simulink model "if_and_if_action_subsys"  (R2014a)
settings: Solver=FixedStepDiscrete  StartTime=0.0  StopTime=10.0  FixedStep=0.1  RelTol=1e-3
settings Model: BufferReuse=off  Creator=yoshi12  LastModifiedBy=ts1413
settings OptimizationCC: BlockReduction=off  OptimizeBlockIOStorage=off  BufferReuse=off  GlobalBufferReuse=off  ExpressionFolding=off  LocalBlockOutputs=off  OptimizeModelRefInitCode=on  LifeSpan=1
settings RTWCC: SystemTargetFile=ert.tlc  GenCodeOnly=on  TemplateMakefile=ert_default_tmf  Description=Embedded Coder  ProcessScript=ert_make_rtw_hook
settings CodeAppCC: IgnoreCustomStorageClasses=off
settings ERTTargetCC: ParMdlRefBuildCompliant=on  CompOptLevelCompliant=on  ConcurrentExecutionCompliant=on  ERTFirstTimeCompliant=on  ModelStepFunctionPrototypeControlCompliant=on  CPPClassGenCompliant=on  InlinedParameterPlacement=Hierarchical  ERTCustomFileTemplate=example_file_process.tlc

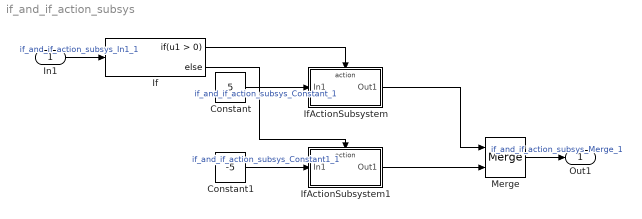
== system if_and_if_action_subsys ==
  In1 : Inport
  Constant : Constant  Value=5
  Constant1 : Constant  Value=-5
  If : If
  IfActionSubsystem : Subsystem  TreatAsAtomicUnit=on
  IfActionSubsystem1 : Subsystem  TreatAsAtomicUnit=on
  Merge : Merge  InitialOutput=0
  Out1 : Outport
  wires:
  In1/1 -> If/1  "if_and_if_action_subsys_In1_1"
  If/1 -> IfActionSubsystem/Action
  If/2 -> IfActionSubsystem1/Action
  IfActionSubsystem/1(Out1) -> Merge/1
  IfActionSubsystem1/1(Out1) -> Merge/2
  Constant/1 -> IfActionSubsystem/1(In1)  "if_and_if_action_subsys_Constant_1"
  Constant1/1 -> IfActionSubsystem1/1(In1)  "if_and_if_action_subsys_Constant1_1"
  Merge/1 -> Out1/1  "if_and_if_action_subsys_Merge_1"

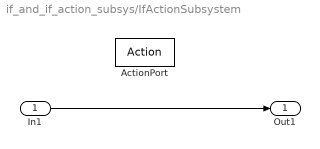
== system if_and_if_action_subsys/IfActionSubsystem ==
  In1 : Inport
  ActionPort : ActionPort  ActionType=then
  Out1 : Outport
  wires:
  In1/1 -> Out1/1

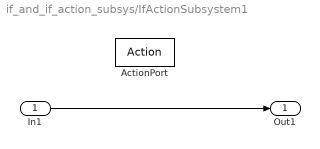
== system if_and_if_action_subsys/IfActionSubsystem1 ==
  In1 : Inport
  ActionPort : ActionPort  ActionType=else
  Out1 : Outport
  wires:
  In1/1 -> Out1/1
